simulink model "ESE4481_hw6_simulink"  (R2021a)
settings: Solver=VariableStepAuto  StartTime=0.0  StopTime=30  RelTol=1e-3
model workspace (MAT data in the model file):
  Kappa = 1
values from neighbouring files (symbols this model uses):
  K_A = place(A_aileron, B_aileron, [-2,-4,-1])    [ESE4481_hw4_poleplacement.m]
  K_E = place(A_elevator, B_elevator, [-2,-4,-1])    [ESE4481_hw4_poleplacement.m]
  K_R = place(A_rudder, B_rudder, [-2,-4])    [ESE4481_hw4_poleplacement.m]
  K_T = place(A_throttle, B_throttle, [-2,-4])    [ESE4481_hw4_poleplacement.m]
undefined symbols (not defined in the file or in its folder): A_a_dis, A_e_dis, A_t_dis, B_a_dis, B_e_dis, B_t_dis, C_a_dis, C_e_dis, C_t_dis, cmd_0, cmd_forward, cmd_hover, coeffs, Discrete, F_aileron, F_elevator, F_rudder, F_throttle, g, J, J_inv, J_p, K_drag, m, M, M_inv, omega_0, p_ned_0, R_t, Theta_0, Time, V_b_0
libraries: vrlib x3, ctrlSharedLib x3, simulink x2
settings Model: Creator=tomwh  LastModifiedBy=tomwh
settings DataIOCC: ExternalInput=F_b,omega_bE,M_b

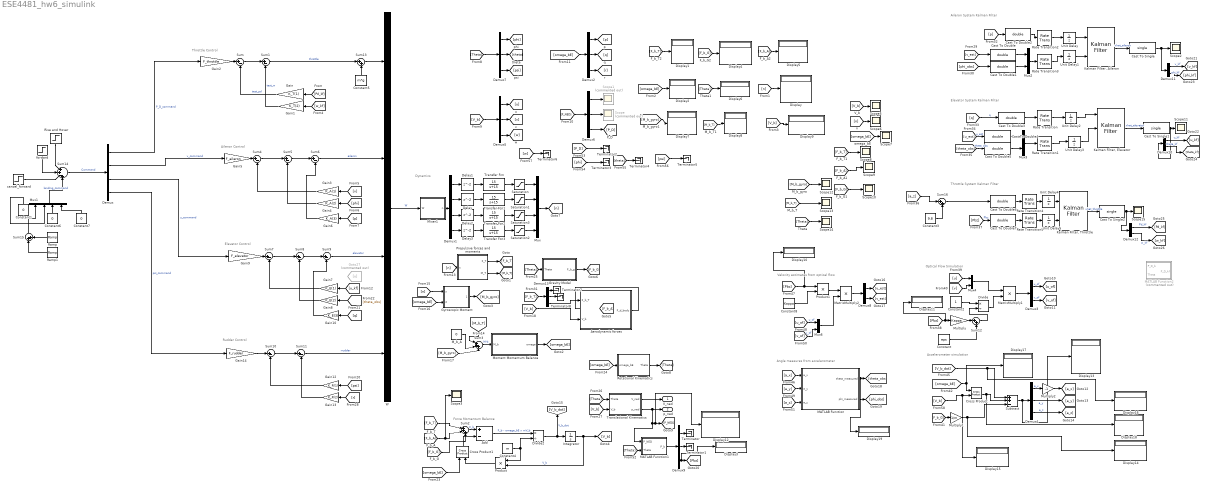
== system ESE4481_hw6_simulink ==
  note: Accelerometer simulation
  note: Force Momentum Balance
  note: Optical Flow Simulation
  note: Rudder Control
  note: Elevator Control
  note: Aileron Control
  note: Throttle Control
  note: Elevator System Kalman Filter
  note: Aileron System Kalman Filter
  note: Throttle System Kalman Filter
  note: Velocity estimates from optical flow
  note: Angle measures from accelerometer
  note: Dynamics
  Add : Sum  Inputs=+-
  Aerodynamic forces : Subsystem
  Cast To Double{,1..7} (8 alike) : DataTypeConversion  OutDataTypeStr=double
  Cast To Single : DataTypeConversion  OutDataTypeStr=single
  Cast To Single1 : DataTypeConversion  OutDataTypeStr=single
  Cast To Single2 : DataTypeConversion  OutDataTypeStr=single
  Constant : Constant  Value=eps
  Constant1 : Constant  Value=0
  Constant2 : Constant
  Constant3 : Constant  Value=9.8
  Constant4 : Constant  Value=m
  Constant5 : Constant  Value=m*g
  Constant6 : Constant  Value=0
  Constant7 : Constant  Value=0
  Constant8 : Constant  Value=Kappa
  Cross Product : vrlib/Utilities/Cross Product
  Cross Product1 : vrlib/Utilities/Cross Product
  Delay{,1..3} (4 alike) : Delay  SampleTime=1/200
  Demux : Demux
  Demux1 : Demux
  Demux{3,8,10..12} (5 alike) : Demux  Outputs=2
  Demux{2,4..7,9,13} (7 alike) : Demux  Outputs=3
  Display{,1..19} (20 alike) : Display
  Divide : Product  Inputs=*/
  Divide2 : Product  Inputs=*/
  Gain : Gain  Gain=K_T(1)
  Gain1 : Gain  Gain=K_T(2)
  Gain10 : Gain  Gain=K_E(3)
  Gain12 : Gain  Gain=K_R(1)
  Gain13 : Gain  Gain=K_R(2)
  Gain14 : Gain  Gain=F_rudder
  Gain2 : Gain  Gain=F_throttle
  Gain3 : Gain  Gain=K_A(1)
  Gain4 : Gain  Gain=K_A(2)
  Gain5 : Gain  Gain=F_aileron
  Gain6 : Gain  Gain=K_A(3)
  Gain7 : Gain  Gain=K_E(1)
  Gain8 : Gain  Gain=K_E(2)
  Gain9 : Gain  Gain=F_elevator
  Goto27 : Goto  Commented=on  GotoTag=u
  Gravity Model : Subsystem
  Gyroscopic Moment : Subsystem
  Integrator : Integrator  InitialCondition=V_b_0
      settings: AttributesFormatString=%<InitialCondition>
  "Kalman Filter, Aileron" : ctrlSharedLib/Kalman Filter  TimeDomain=Discrete-Time  UseCurrentEstimator=on  ModelSource=Individual A, B, C, D matrices  ModelSourceVariable=ss(0.95,1,1,0,1)  A=A_a_dis  B=B_a_dis  C=C_a_dis  D=[0;0]  NumberOfStates=1  NumberOfInputs=1  NumberOfOutputs=1  InitialEstimateSource=Dialog  X0=[0;0]  P0=10  UseK=off  UseGH=off  NumberOfProcessNoiseInputs=1  G=1  TimeInvariantG=on  H=0  TimeInvariantH=on  Q=Q_a_dis  TimeInvariantQ=on  R=eye(2)  TimeInvariantR=on  N=0  TimeInvariantN=on  AddInputPort=on  AddEnablePort=off  OutputEstimatedY=off  OutputP=off  Ts=1/200
  "Kalman Filter, Elevator" : ctrlSharedLib/Kalman Filter  TimeDomain=Discrete-Time  UseCurrentEstimator=on  ModelSource=Individual A, B, C, D matrices  ModelSourceVariable=ss(0.95,1,1,0,1)  A=A_e_dis  B=B_e_dis  C=C_e_dis  D=[0]  NumberOfStates=1  NumberOfInputs=1  NumberOfOutputs=1  InitialEstimateSource=Input port  X0=0  P0=10  UseK=off  UseGH=off  NumberOfProcessNoiseInputs=1  G=1  TimeInvariantG=on  H=0  TimeInvariantH=on  Q=Q_e_dis  TimeInvariantQ=on  R=[1/50 0; 0 1]  TimeInvariantR=on  N=0  TimeInvariantN=on  AddInputPort=on  AddEnablePort=off  OutputEstimatedY=off  OutputP=off  Ts=1/200
  "Kalman Filter, Throttle" : ctrlSharedLib/Kalman Filter  TimeDomain=Discrete-Time  UseCurrentEstimator=on  ModelSource=Individual A, B, C, D matrices  ModelSourceVariable=ss(0.95,1,1,0,1)  A=A_t_dis  B=B_t_dis  C=C_t_dis  D=0  NumberOfStates=1  NumberOfInputs=1  NumberOfOutputs=1  InitialEstimateSource=Dialog  X0=0  P0=10  UseK=off  UseGH=off  NumberOfProcessNoiseInputs=1  G=1  TimeInvariantG=on  H=0  TimeInvariantH=on  Q=Q_t_dis  TimeInvariantQ=on  R=R_t  TimeInvariantR=on  N=0  TimeInvariantN=on  AddInputPort=on  AddEnablePort=off  OutputEstimatedY=off  OutputP=off  Ts=1/200
  MATLAB Function : MATLAB Function  TreatAsAtomicUnit=on
  MATLAB Function1 : MATLAB Function  TreatAsAtomicUnit=on
  MATLAB Function2 : MATLAB Function  Commented=on  TreatAsAtomicUnit=on
  M_b_A : Constant  Value=0
  MatrixMultiply1 : Product
  MatrixMultiply2 : Product
  Mixer1 : Subsystem
  Moment Momentum Balance : Subsystem
  Multiply : Gain  Gain=Kappa
  Multiply1 : Gain  Gain=1/m
  Multiply2 : Gain  Gain=-1
  Mux : Mux
  Mux1 : Mux
  Mux{2..4,6} (4 alike) : Mux  Inputs=2
  Product : Product
  Product1 : Product
  Propulsive forces and moments : Subsystem
  Ramp : simulink/Sources/Ramp  slope=.2  start=21  InitialOutput=0
  Ramp1 : simulink/Sources/Ramp  slope=-.2  start=26  InitialOutput=0
  Rate Transition{,1..5} (6 alike) : RateTransition  OutPortSampleTime=dt
  Rise and Hover : Step  Before=cmd_0  After=cmd_hover  SampleTime=0
  Rotational Kinematics : Subsystem
  Saturation{,1..3} (4 alike) : Saturate  UpperLimit=500  LowerLimit=0
  Scope : Scope  Commented=on
  Scope1 : Scope  Commented=on
  Scope{2..3,5..15} (13 alike) : Scope
  Subtract : Sum  Inputs=++-
  Sum{,1,4..11} (10 alike) : Sum  Inputs=|+-
  Sum{12..13,15..16} (4 alike) : Sum  Inputs=|++
  Sum14 : Sum  Inputs=|++-+
  Sum2 : Sum  Inputs=|+++
  Sum3 : Sum  Inputs=|+++
  Terminator{,1..8} (9 alike) : Terminator
  Transfer Fcn{,1..3} (4 alike) : TransferFcn  Numerator=[15]  Denominator=[1 15]
  Translational Kinematics : Subsystem
  Unit Delay{,1..5} (6 alike) : UnitDelay  SampleTime=1/200  HasFrameUpgradeWarning=on
  W : Mux
  cancel_forward : Step  Time=16  After=cmd_forward  SampleTime=0
  forward : Step  Time=6  After=cmd_forward  SampleTime=0
  V_ned : Outport
  p_ned : Outport  Port=2
  wires:
  [V_b] -> Scope5/1
  [n] -> Scope6/1
  [omega_bE] -> Scope7/1
  [F_b_T] -> Scope8/1
  [Theta] -> Scope14/1
  [M_b_T] -> Scope13/1
  [M_b_gyro] -> Scope12/1
  [F_b_G] -> Scope10/1
  [F_b_A] -> Scope9/1
  [n] -> Display/1
  [F_b_T] -> Display1/1
  [omega_bE] -> Display2/1
  [F_b_G] -> Display4/1
  [F_b_A] -> Display5/1
  [Theta] -> Display6/1
  [M_b_gyro] -> Display7/1
  [M_b_T] -> Display8/1
  [V_b] -> Display9/1
  Translational Kinematics/1(V_ned) -> V_ned/1
  Demux1/1 -> Delay1/1
  Saturation3/1 -> Mux/3
  Transfer Fcn2/1 -> Saturation3/1
  Saturation1/1 -> Mux/2
  Saturation2/1 -> Mux/4
  Saturation/1 -> Mux/1
  Transfer Fcn3/1 -> Saturation2/1
  Demux1/4 -> Delay3/1
  Delay3/1 -> Transfer Fcn3/1
  Demux1/3 -> Delay2/1
  Delay2/1 -> Transfer Fcn2/1
  Transfer Fcn1/1 -> Saturation1/1
  Demux1/2 -> Delay/1
  Delay/1 -> Transfer Fcn1/1
  Transfer Fcn/1 -> Saturation/1
  Delay1/1 -> Transfer Fcn/1
  [Theta] -> Gravity Model/1(Theta)
  M_b_A/1 -> Sum3/2
  Mixer1/1(n) -> Demux1/1
  Propulsive forces and moments/1(F_T) -> [F_b_T]
  Rotational Kinematics/1(Theta) -> [Theta]
  [Theta] -> Translational Kinematics/1(Theta)
  Propulsive forces and moments/2(M_T) -> [M_b_T]
  Gyroscopic Moment/1(M_gyro) -> [M_b_gyro]
  [n] -> Propulsive forces and moments/1(n)
  [F_b_G] -> Sum2/3
  [n] -> Gyroscopic Moment/1(n)
  [omega_bE] -> Gyroscopic Moment/2(omega_bE)
  [M_b_gyro] -> Sum3/3
  Sum3/1 -> Moment Momentum Balance/1(M_b)  "M-b"
  [M_b_T] -> Sum3/1
  [F_b_A] -> Scope3/1, Sum2/2
  Sum2/1 -> Add/1  "F_b"
  [F_b_T] -> Sum2/1
  W/1 -> Mixer1/1(W)  "W"
  [omega_bE] -> Rotational Kinematics/1(omega_bE)
  Moment Momentum Balance/1(omega) -> [omega_bE]
  [V_b] -> Translational Kinematics/2(V_b)
  Sum/1 -> Sum1/1
  Gain1/1 -> Sum1/2  "test_w"
  [Pd_kf] -> Gain/1
  Gain/1 -> Sum/2  "test_pd"
  Gain2/1 -> Sum/1
  [w_kf] -> Gain1/1
  Demux/1 -> Gain2/1  "P_D_command"
  Demux7/3 -> [psi]
  Demux7/2 -> [theta]
  Demux5/3 -> [w]
  Demux5/1 -> [u]
  Demux5/2 -> [v]
  Demux7/1 -> [phi]
  [Theta] -> Demux7/1
  [V_b] -> Demux5/1
  [P_NED] -> Demux6/1
  Demux2/3 -> [r]
  [omega_bE] -> Demux2/1
  Demux2/1 -> [p]
  Demux2/2 -> [q]
  Demux/2 -> Gain5/1  "v_command"
  Sum5/1 -> Sum6/1
  Sum4/1 -> Sum5/1
  Gain6/1 -> Sum6/2
  [phi] -> Gain4/1
  Gain5/1 -> Sum4/1
  Gain4/1 -> Sum5/2
  [p] -> Gain6/1
  [v] -> Gain3/1
  Gain3/1 -> Sum4/2
  Demux/3 -> Gain9/1  "u_command"
  [u_kf] -> Gain7/1
  Gain8/1 -> Sum8/2
  [q] -> Gain10/1
  Gain10/1 -> Sum9/2
  Gain9/1 -> Sum7/1
  Gain7/1 -> Sum7/2
  Sum7/1 -> Sum8/1
  Sum9/1 -> W/3  "elevator"
  [theta_obs] -> Gain8/1
  Sum8/1 -> Sum9/1
  Demux/4 -> Gain14/1  "psi_command"
  [psi] -> Gain12/1
  Sum11/1 -> W/4  "rrudder"
  Gain12/1 -> Sum10/2
  Gain14/1 -> Sum10/1
  Sum10/1 -> Sum11/1
  Gain13/1 -> Sum11/2
  [r] -> Gain13/1
  Sum13/1 -> W/1
  Demux6/3 -> [P_D]
  Demux6/2 -> Scope/1
  Demux6/1 -> Scope1/1
  Sum14/1 -> Demux/1  "Command"
  Rise and Hover/1 -> Sum14/1
  forward/1 -> Sum14/2
  cancel_forward/1 -> Sum14/3
  Sum1/1 -> Sum13/1  "throttle"
  Constant5/1 -> Sum13/2
  Mux/1 -> [n]
  Sum6/1 -> W/2  "aileron"
  Ramp/1 -> Sum15/2
  Ramp1/1 -> Sum15/1
  Mux1/1 -> Sum14/4  "landing_command"
  Sum15/1 -> Mux1/1
  Constant1/1 -> Mux1/2
  Constant6/1 -> Mux1/3
  Constant7/1 -> Mux1/4
  Aerodynamic forces/1(F_d_body) -> [F_b_A]
  Translational Kinematics/2(p_ned) -> MATLAB Function1/1(P_NED), Display12/1, [P_NED], p_ned/1
  Gravity Model/1(F_b_g) -> [F_b_G]
  Cast To Double4/1 -> Mux3/1
  Cast To Double5/1 -> Mux3/2
  Cast To Double3/1 -> Rate Transition/1
  "Kalman Filter, Elevator"/1 -> Cast To Single1/1  "xhat_elevator"
  Mux3/1 -> Rate Transition1/1
  [u_est] -> Cast To Double4/1  "u_est"
  [q] -> Cast To Double3/1  "q"
  [theta_obs] -> Cast To Double5/1  "theta_obs"
  Cast To Single1/1 -> Demux10/1, Scope11/1
  "Kalman Filter, Aileron"/1 -> Cast To Single/1  "xhat_aileron"
  [v_est] -> Cast To Double/1
  Mux2/1 -> Rate Transition3/1
  Cast To Double1/1 -> Mux2/2
  Cast To Double/1 -> Mux2/1
  [phi_obs] -> Cast To Double1/1
  [p] -> Cast To Double2/1
  Cast To Double2/1 -> Rate Transition2/1
  Cast To Single/1 -> Demux11/1, Scope2/1
  "Kalman Filter, Throttle"/1 -> Cast To Single2/1  "xhat_throttle"
  Cast To Double7/1 -> Rate Transition5/1
  [Pbz] -> Cast To Double7/1  "Pbz"
  Cast To Double6/1 -> Rate Transition4/1
  Cast To Single2/1 -> Demux12/1, Scope15/1
  [u] -> Mux4/1
  [v] -> Mux4/2
  Constant2/1 -> Divide/1
  MatrixMultiply1/1 -> Demux3/1
  Demux3/1 -> [u_of]  "u_of"
  Demux3/2 -> [v_of]  "v_of"
  Unit Delay2/1 -> "Kalman Filter, Elevator"/1
  Rate Transition/1 -> Unit Delay2/1
  Unit Delay3/1 -> "Kalman Filter, Elevator"/2
  Rate Transition1/1 -> Unit Delay3/1
  Rate Transition4/1 -> Unit Delay4/1
  Unit Delay4/1 -> "Kalman Filter, Throttle"/1
  Rate Transition5/1 -> Unit Delay5/1
  Unit Delay5/1 -> "Kalman Filter, Throttle"/2
  Unit Delay/1 -> "Kalman Filter, Aileron"/1
  Rate Transition2/1 -> Unit Delay/1
  Rate Transition3/1 -> Unit Delay1/1
  Unit Delay1/1 -> "Kalman Filter, Aileron"/2
  Product/1 -> Cross Product1/2
  Cross Product1/1 -> Add/2
  Add/1 -> Divide2/1  "F_b - omega_bE x mV_b"
  Divide2/1 -> [V_b_dot], Integrator/1  "V_b_dot"
  Constant4/1 -> Divide2/2, Product/1
  Integrator/1 -> Product/2, [V_b]  "V_b"
  [omega_bE] -> Cross Product1/1
  Mux4/1 -> MatrixMultiply1/1
  Divide/1 -> MatrixMultiply1/2
  Demux8/1 -> [u_est]
  MATLAB Function/1(theta_measured) -> Display19/1, [theta_obs]
  MATLAB Function/2(phi_measured) -> [phi_obs]
  [Pbz] -> Display10/1, Product1/1
  [a_z] -> MATLAB Function/3(a_z)
  Constant8/1 -> Product1/2
  [v_of] -> Mux6/2  "v_of"
  Mux6/1 -> MatrixMultiply2/2
  [a_x] -> MATLAB Function/1(a_x)
  Product1/1 -> MatrixMultiply2/1
  [u_of] -> Mux6/1  "u_of"
  Demux8/2 -> [v_est]
  [a_y] -> MATLAB Function/2(a_y)
  MatrixMultiply2/1 -> Demux8/1
  [Theta] -> MATLAB Function1/2(Theta)
  MATLAB Function1/1(P_b) -> Demux9/1
  Demux9/1 -> Terminator/1
  Demux9/2 -> Terminator1/1
  Demux9/3 -> Display3/1, [Pbz]
  Demux4/3 -> [a_z]  "a_z"
  Demux4/1 -> Multiply2/1  "a_x"
  Demux4/2 -> [a_y]  "a_y"
  Demux11/1 -> [v_kf]  "v_kf"
  Demux11/2 -> [phi_kf]  "phi_kf"
  Demux10/1 -> [u_kf]  "u_kf"
  Demux12/1 -> [Pd_kf]  "Pd_kf"
  Demux12/2 -> [w_kf]  "w_kf"
  [P_D] -> Terminator2/1
  [phi] -> Terminator3/1
  [theta] -> Terminator4/1
  [psi] -> Terminator5/1
  [w] -> Terminator6/1
  [Pbz] -> Display11/1, Multiply/1
  Multiply/1 -> Sum12/1
  Constant/1 -> Sum12/2
  Sum12/1 -> Divide/2
  [V_b] -> Display15/1, Cross Product/2
  Cross Product/1 -> Display18/1, Subtract/2
  [V_b_dot] -> Display16/1, Subtract/1
  [omega_bE] -> Cross Product/1, Display17/1
  Subtract/1 -> Display13/1, Demux4/1
  [F_b_G] -> Multiply1/1
  Multiply1/1 -> Display14/1, Subtract/3
  [V_b] -> Aerodynamic forces/2(V_b)
  [a_z] -> Sum16/1
  Constant3/1 -> Sum16/2
  Sum16/1 -> Cast To Double6/1
  Demux10/2 -> [theta_kf]  "theta_kf"
  [F_b_T] -> Demux13/1
  Demux13/1 -> Terminator7/1
  Demux13/2 -> Terminator8/1
  Demux13/3 -> Aerodynamic forces/1(F_b_T)
  Multiply2/1 -> [a_x]

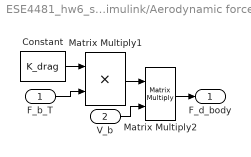
== system ESE4481_hw6_simulink/Aerodynamic forces ==
  F_b_T : Inport
  V_b : Inport  Port=2
  Constant : Constant  Value=K_drag
  Matrix Multiply1 : Product
  Matrix Multiply2 : Product  Multiplication=Matrix(*)
  F_d_body : Outport
  wires:
  V_b/1 -> Matrix Multiply2/2
  Matrix Multiply2/1 -> F_d_body/1
  Matrix Multiply1/1 -> Matrix Multiply2/1
  Constant/1 -> Matrix Multiply1/1
  F_b_T/1 -> Matrix Multiply1/2

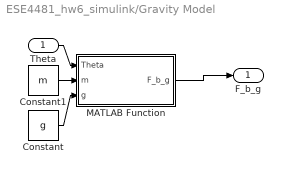
== system ESE4481_hw6_simulink/Gravity Model ==
  Theta : Inport
  Constant : Constant  Value=g
  Constant1 : Constant  Value=m
  MATLAB Function : MATLAB Function  TreatAsAtomicUnit=on
  F_b_g : Outport
  wires:
  Theta/1 -> MATLAB Function/1(Theta)
  MATLAB Function/1(F_b_g) -> F_b_g/1
  Constant/1 -> MATLAB Function/3(g)
  Constant1/1 -> MATLAB Function/2(m)

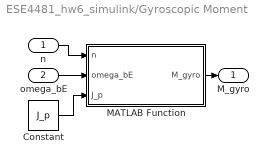
== system ESE4481_hw6_simulink/Gyroscopic Moment ==
  n : Inport
  omega_bE : Inport  Port=2
  Constant : Constant  Value=J_p
  MATLAB Function : MATLAB Function  TreatAsAtomicUnit=on
  M_gyro : Outport
  wires:
  n/1 -> MATLAB Function/1(n)
  MATLAB Function/1(M_gyro) -> M_gyro/1
  omega_bE/1 -> MATLAB Function/2(omega_bE)
  Constant/1 -> MATLAB Function/3(J_p)

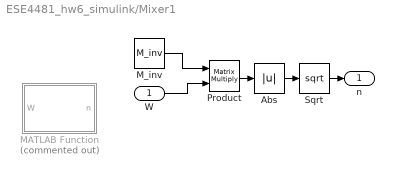
== system ESE4481_hw6_simulink/Mixer1 ==
  W : Inport
  Abs : Abs
  MATLAB Function : MATLAB Function  Commented=on  TreatAsAtomicUnit=on
  M_inv : Constant  Value=M_inv
  Product : Product  Multiplication=Matrix(*)
  Sqrt : Sqrt  SaturateOnIntegerOverflow=on
  n : Outport
  wires:
  M_inv/1 -> Product/1
  W/1 -> Product/2
  Product/1 -> Abs/1
  Abs/1 -> Sqrt/1
  Sqrt/1 -> n/1

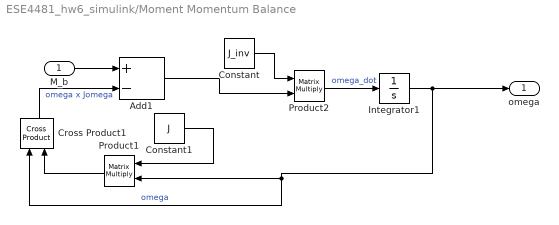
== system ESE4481_hw6_simulink/Moment Momentum Balance ==
  M_b : Inport
  Add1 : Sum  Inputs=+-
  Constant : Constant  Value=J_inv
  Constant1 : Constant  Value=J
  Cross Product1 : vrlib/Utilities/Cross Product
  Integrator1 : Integrator  InitialCondition=omega_0
      settings: AttributesFormatString=%<InitialCondition>
  Product1 : Product  Multiplication=Matrix(*)
  Product2 : Product  Multiplication=Matrix(*)
  omega : Outport
  wires:
  Constant1/1 -> Product1/1
  Cross Product1/1 -> Add1/2  "omega x Jomega"
  Integrator1/1 -> omega/1, Cross Product1/1, Product1/2  "omega"
  Product1/1 -> Cross Product1/2
  Product2/1 -> Integrator1/1  "omega_dot"
  M_b/1 -> Add1/1
  Constant/1 -> Product2/1
  Add1/1 -> Product2/2

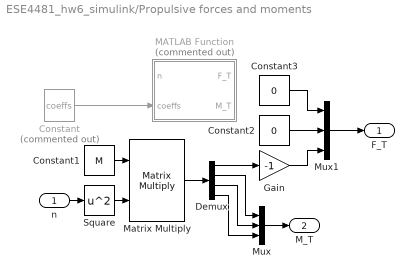
== system ESE4481_hw6_simulink/Propulsive forces and moments ==
  n : Inport
  Constant : Constant  Commented=on  Value=coeffs
  Constant1 : Constant  Value=M
  Constant2 : Constant  Value=0
  Constant3 : Constant  Value=0
  Demux : Demux
  Gain : Gain  Gain=-1
  MATLAB Function : MATLAB Function  Commented=on  TreatAsAtomicUnit=on
  Matrix Multiply : Product  Multiplication=Matrix(*)
  Mux : Mux  Inputs=3
  Mux1 : Mux  Inputs=3
  Square : Math  Operator=square  SaturateOnIntegerOverflow=on
  F_T : Outport
  M_T : Outport  Port=2
  wires:
  Constant/1 -> MATLAB Function/2(coeffs)
  Constant1/1 -> Matrix Multiply/1
  Matrix Multiply/1 -> Demux/1
  Demux/2 -> Mux/1
  Demux/3 -> Mux/2
  Demux/4 -> Mux/3
  Square/1 -> Matrix Multiply/2
  Demux/1 -> Gain/1
  n/1 -> Square/1
  Constant3/1 -> Mux1/1
  Constant2/1 -> Mux1/2
  Gain/1 -> Mux1/3
  Mux1/1 -> F_T/1
  Mux/1 -> M_T/1

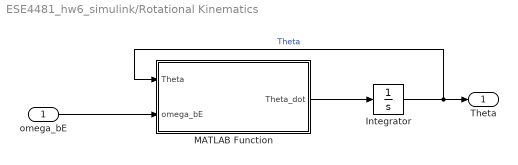
== system ESE4481_hw6_simulink/Rotational Kinematics ==
  omega_bE : Inport
  Integrator : Integrator  InitialCondition=Theta_0
      settings: AttributesFormatString=%<InitialCondition>
  MATLAB Function : MATLAB Function  TreatAsAtomicUnit=on
  Theta : Outport
  wires:
  Integrator/1 -> MATLAB Function/1(Theta), Theta/1  "Theta"
  omega_bE/1 -> MATLAB Function/2(omega_bE)
  MATLAB Function/1(Theta_dot) -> Integrator/1

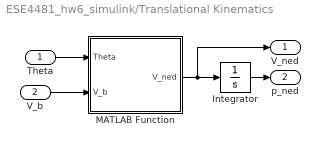
== system ESE4481_hw6_simulink/Translational Kinematics ==
  Theta : Inport
  V_b : Inport  Port=2
  Integrator : Integrator  InitialCondition=p_ned_0
      settings: AttributesFormatString=%<InitialCondition>
  MATLAB Function : MATLAB Function  TreatAsAtomicUnit=on
  V_ned : Outport
  p_ned : Outport  Port=2
  wires:
  MATLAB Function/1(V_ned) -> V_ned/1, Integrator/1
  V_b/1 -> MATLAB Function/2(V_b)
  Integrator/1 -> p_ned/1
  Theta/1 -> MATLAB Function/1(Theta)

== matlab function ESE4481_hw6_simulink/MATLAB Function1 ==
  data: P_NED input; P_b output; Theta input
function P_b = fcn(P_NED,Theta)
    phi = Theta(1);
    theta = Theta(2);
    psi = Theta(3);
    R_phi = [1 0 0;
             0 cos(phi) sin(phi);
             0 -sin(phi) cos(phi)];
    R_theta = [cos(theta) 0 -sin(theta);
               0 1 0;
               sin(theta) 0 cos(theta)];
    R_psi = [cos(psi) sin(psi) 0;
             -sin(psi) cos(psi) 0;
             0 0 1];
    R_b_E = R_phi*R_theta*R_psi;
    P_b = R_b_E*P_NED;

== matlab function ESE4481_hw6_simulink/MATLAB Function ==
  data: a_x input; theta_measured output; a_y input; a_z input; phi_measured output
function [theta_measured,phi_measured]= fcn(a_x,a_y,a_z)
theta_measured = -a_x / sqrt(a_y^2 + a_z^2+ eps);
phi_measured = a_y/(a_z+eps);
%conditional logic here, safe division

== matlab function ESE4481_hw6_simulink/MATLAB Function2 ==
  data: P_D_b input; P_D_kf output; Theta input
function P_D_kf = fcn(P_D_b,Theta)
    phi = Theta(1);
    theta = Theta(2);
    psi = Theta(3);
    P_b = [0 0 P_D_b]';
    R_phi = [1 0 0;
             0 cos(phi) sin(phi);
             0 -sin(phi) cos(phi)];
    R_theta = [cos(theta) 0 -sin(theta);
               0 1 0;
               sin(theta) 0 cos(theta)];
    R_psi = [cos(psi) sin(psi) 0;
             -sin(psi) cos(psi) 0;
             0 0 1];
    R_b_E = R_phi*R_theta*R_psi;
    P_NED = R_b_E*P_b;
    P_D_kf = P_NED(3);

== matlab function ESE4481_hw6_simulink/Mixer1/MATLAB Function ==
  data: W input; n output
function n = getMotorSpeeds(W)
% a = 2.034763500512882e-06;
% b = 9.690561171192599e-08;
% c = b;
% d = 1.056628184682481e-08;
rho = 1.293;
D = 0.066;
C_t = @(n) 4.375*10^(-5)*n + 0.0704; 
C_p = 0.041;
dist_xy = 0.047625; 
n_eq = 2.893014369037372e+02;
a = C_t(n_eq)*rho*D^4;
b = C_t(n_eq)*rho*D^4*dist_xy;
c = b;
d = C_p*rho*D^5/(2*pi);
M = [a a a a;
    b -b -b b;
    c c -c -c;
    -d d -d d];
nu = abs(M\W);
n = sqrt(nu);

== matlab function ESE4481_hw6_simulink/Propulsive forces and moments/MATLAB Function ==
  data: n input; F_T output; M_T output; coeffs input
function [F_T,M_T]= fcn(n,coeffs)
a = coeffs(1);
b = coeffs(2);
c = coeffs(3);
d = coeffs(4);
% Wrench = M*[n(1)^2; n(2)^2; n(3)^2; n(4)^2];
F_T = [0;0; -a*(n(1)^2 + n(2)^2 + n(3)^2 + n(4)^2)];
M_T = [b*(n(1)^2 - n(2)^2 - n(3)^2 + n(4)^2); c*(n(1)^2 + n(2)^2 - n(3)^2 - n(4)^2); d*(-n(1)^2 + n(2)^2 - n(3)^2 + n(4)^2)];
% F_T = Wrench(1);
% M_T = Wrench(2:4);

== matlab function ESE4481_hw6_simulink/Gyroscopic Moment/MATLAB Function ==
  data: n input; M_gyro output; omega_bE input; J_p input
function M_gyro = fcn(n,omega_bE,J_p)
    H = [0;0; J_p*2*pi*(n(1)-n(2)+n(3)-n(4))];
M_gyro = cross(omega_bE,H);

== matlab function ESE4481_hw6_simulink/Gravity Model/MATLAB Function ==
  data: Theta input; F_b_g output; m input; g input
function F_b_g = fcn(Theta,m,g)
phi = Theta(1);
theta = Theta(2);
psi = Theta(3);
R_phi = [1 0 0;
         0 cos(phi) sin(phi);
         0 -sin(phi) cos(phi)];
R_theta = [cos(theta) 0 -sin(theta);
           0 1 0;
           sin(theta) 0 cos(theta)];
R_psi = [cos(psi) sin(psi) 0;
         -sin(psi) cos(psi) 0;
         0 0 1];
R_b_E = R_phi*R_theta*R_psi;
F_b_g = R_b_E*[0; 0; m*g];

== matlab function ESE4481_hw6_simulink/Rotational Kinematics/MATLAB Function ==
  data: Theta input; Theta_dot output; omega_bE input
function Theta_dot = fcn(Theta,omega_bE)
    phi = Theta(1);
    theta = Theta(2);
    H_inv = [1 sin(phi)*tan(theta) cos(phi)*tan(theta);
             0 cos(phi) -sin(phi);
             0 sin(phi)*sec(theta) cos(phi)*sec(theta)];
Theta_dot = H_inv*omega_bE;

== matlab function ESE4481_hw6_simulink/Translational Kinematics/MATLAB Function ==
  data: Theta input; V_ned output; V_b input
function V_ned = fcn(Theta,V_b)
phi = Theta(1);
theta = Theta(2);
psi = Theta(3);
% R_phi = [1 0 0;
%          0 cos(phi) sin(phi);
%          0 -sin(phi) cos(phi)];
% R_theta = [cos(theta) 0 -sin(theta);
%            0 1 0;
%            sin(theta) 0 cos(theta)];
% R_psi = [cos(psi) sin(psi) 0;
%          -sin(psi) cos(psi) 0;
%          0 0 1];
% R = R_phi*R_theta*R_psi;
R = [cos(psi)*cos(theta) cos(theta)*sin(psi) -sin(theta);
     cos(psi)*sin(phi)*sin(theta)-cos(phi)*sin(psi) cos(phi)*cos(psi)+sin(phi)*sin(psi)*sin(theta) cos(theta)*sin(phi)
     sin(phi)*sin(psi)+cos(phi)*cos(psi)*sin(theta) cos(phi)*sin(psi)*sin(theta)-cos(psi)*sin(phi) cos(phi)*cos(theta)];
V_ned = R\V_b; %\V_b
